simulink model "control_lab2"  (R2022b)
settings: Solver=VariableStepAuto  StartTime=0.0  StopTime=10.0  RelTol=1e-3
settings Model: Creator=Asus  LastModifiedBy=Asus

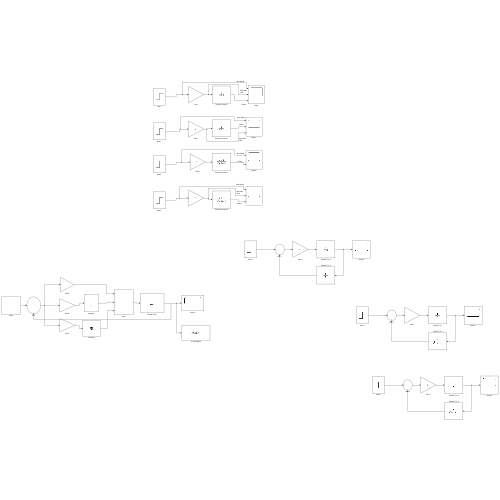
[thumbnail: Simulink's stored preview of the top-level diagram]
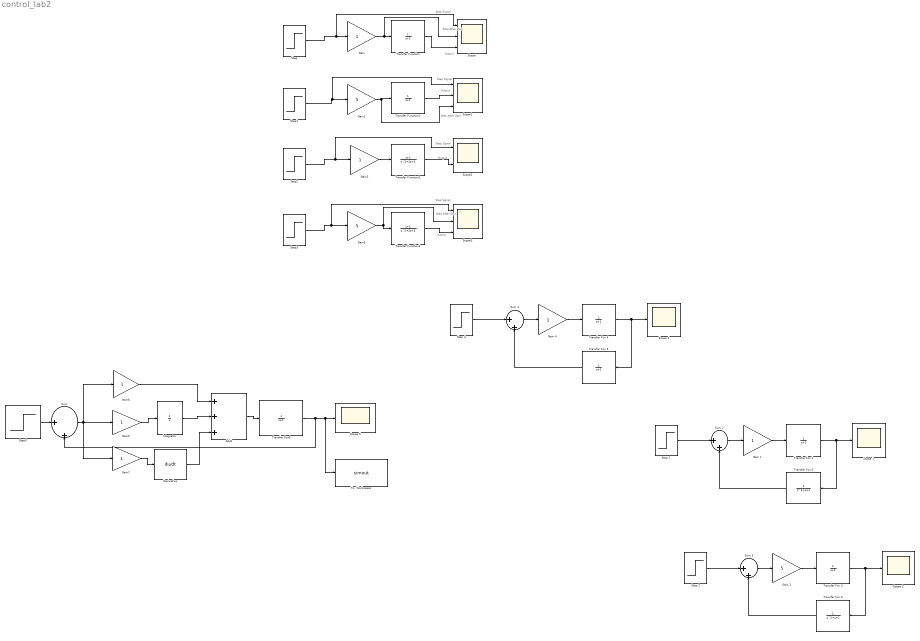
== system control_lab2 ==
  note: Output
  note: Step Signal
  note: Step After
      | Gain
  note: Step Signal
  note: Step After
      | Gain
  note: Output
  note: Step Signal
  note: Output
  note: Output
  note: Step Signal
  note: Step After
      | Gain
  "Add1 " : Sum  Inputs=+++
  "Derivative " : Derivative
  "Gain " : Gain
  Gain 1 : Gain
  Gain 2 : Gain  Gain=5
  Gain 4 : Gain
  "Gain1 " : Gain  Gain=5
  "Gain2 " : Gain
  Gain3 : Gain  Gain=5
  "Gain5 " : Gain
  "Gain6 " : Gain
  "Gain7 " : Gain
  "Integrator " : Integrator
  "Scope " : Scope  NumInputPorts=3
  Scope {1..2,4..5} (4 alike) : Scope
  "Scope1 " : Scope  NumInputPorts=3
  "Scope2 " : Scope  NumInputPorts=2
  Scope3 : Scope  NumInputPorts=3
  Step {,1..2,4} (4 alike) : Step  SampleTime=0
  "Step1 " : Step  SampleTime=0
  "Step2 " : Step  SampleTime=0
  "Step3 " : Step  SampleTime=0
  "Step5 " : Step  SampleTime=0
  Sum {,1..3} (4 alike) : Sum  Inputs=|++
  To  Workspace : ToWorkspace  VariableName=simout  SaveFormat=Timeseries  SampleTime=-1
  Transfer Fcn {1,3..5} (4 alike) : TransferFcn  Denominator=[1 1]
  Transfer Fcn 2 : TransferFcn  Denominator=[1 1 1]
  Transfer Fcn 6 : TransferFcn  Denominator=[1 1 1]
  "Transfer Fcn6 " : TransferFcn  Denominator=[1 1]
  Transfer Function : TransferFcn  Denominator=[1 1]
  Transfer Function1 : TransferFcn  Denominator=[1 1]
  "Transfer Function2 " : TransferFcn  Numerator=[1 1]  Denominator=[1 2 3]
  Transfer Function3 : TransferFcn  Numerator=[1 1]  Denominator=[1 2 3]
  wires:
  "Gain "/1 -> "Scope "/2, Transfer Function/1
  "Step "/1 -> "Scope "/1, "Gain "/1
  "Gain1 "/1 -> "Scope1 "/3, Transfer Function1/1
  Transfer Function1/1 -> "Scope1 "/2
  "Step1 "/1 -> "Scope1 "/1, "Gain1 "/1
  Gain3/1 -> Transfer Function3/1, Scope3/2
  "Step3 "/1 -> Scope3/1, Gain3/1
  Transfer Function3/1 -> Scope3/3
  "Gain2 "/1 -> "Transfer Function2 "/1
  "Step2 "/1 -> "Scope2 "/1, "Gain2 "/1
  "Transfer Function2 "/1 -> "Scope2 "/2
  Transfer Fcn 4/1 -> Transfer Fcn 5/1, Scope 4/1
  Gain 4/1 -> Transfer Fcn 4/1
  "Step5 "/1 -> "Sum "/1
  "Sum "/1 -> "Gain6 "/1, "Gain7 "/1, "Gain5 "/1
  "Gain5 "/1 -> "Integrator "/1
  "Gain7 "/1 -> "Derivative "/1
  "Gain6 "/1 -> "Add1 "/1
  "Integrator "/1 -> "Add1 "/2
  "Derivative "/1 -> "Add1 "/3
  "Add1 "/1 -> "Transfer Fcn6 "/1
  "Transfer Fcn6 "/1 -> Scope 5/1, To  Workspace/1, "Sum "/2
  Step 4/1 -> Sum 1/1
  Sum 1/1 -> Gain 4/1
  Transfer Function/1 -> "Scope "/3
  Transfer Fcn 5/1 -> Sum 1/2
  Transfer Fcn 2/1 -> Sum 2/2
  Step 1/1 -> Sum 2/1
  Transfer Fcn 1/1 -> Transfer Fcn 2/1, Scope 1/1
  Sum 2/1 -> Gain 1/1
  Gain 1/1 -> Transfer Fcn 1/1
  Gain 2/1 -> Transfer Fcn 3/1
  Step 2/1 -> Sum 3/1
  Transfer Fcn 6/1 -> Sum 3/2
  Sum 3/1 -> Gain 2/1
  Transfer Fcn 3/1 -> Transfer Fcn 6/1, Scope 2/1
